simulink model "p2a"  (R2017b)
settings: Solver=FixedStepAuto  StartTime=0.0  StopTime=10.0  FixedStep=0.01  RelTol=1e-3
values from neighbouring files (symbols this model uses):
  a = [ -0.0000 1.0000 -0.0000 -0.0000 ... (first row only)    [observer.m]    (also in p2a.m)
  b = [ -0.0000 0.0000 ... (first row only)    [observer.m]    (also in p2a.m)
  c = [ 1.0000 -0.0050 0.0000 0.0000 ... (first row only)    [observer.m]    (also in p2a.m)
undefined symbols (not defined in the file or in its folder): K, l1
settings Model: Creator=Soutrik  LastModifiedBy=Soutrik

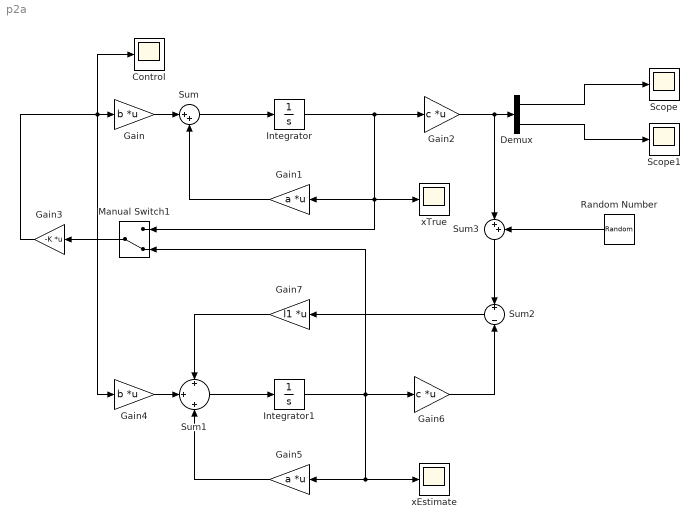
== system p2a ==
  Control : Scope
  Demux : Demux  Outputs=2
  Gain : Gain  Gain=b  Multiplication=Matrix(K*u)
  Gain1 : Gain  Gain=a  Multiplication=Matrix(K*u)
  Gain2 : Gain  Gain=c  Multiplication=Matrix(K*u)
  Gain3 : Gain  Gain=-K  Multiplication=Matrix(K*u)
  Gain4 : Gain  Gain=b  Multiplication=Matrix(K*u)
  Gain5 : Gain  Gain=a  Multiplication=Matrix(K*u)
  Gain6 : Gain  Gain=c  Multiplication=Matrix(K*u)
  Gain7 : Gain  Gain=l1  Multiplication=Matrix(K*u)
  Integrator : Integrator  InitialCondition=[0.05, 0, 0, 0]
  Integrator1 : Integrator  InitialCondition=[0.05, 0, 0, 0]
  Manual Switch1 : ManualSwitch  CurrentSetting=0
  Random Number : RandomNumber  Variance=[0.00001, 0.00001, 0.0001, 0.0001]  Seed=[1 2 3 4]  SampleTime=0.01
  Scope : Scope
  Scope1 : Scope
  Sum : Sum  Inputs=|++
  Sum1 : Sum  Inputs=+|+|+
  Sum2 : Sum  Inputs=+||-
  Sum3 : Sum  Inputs=|++
  xEstimate : Scope
  xTrue : Scope
  wires:
  Random Number/1 -> Sum3/2
  Gain7/1 -> Sum1/1
  Sum3/1 -> Sum2/1
  Manual Switch1/1 -> Gain3/1
  Gain2/1 -> Sum3/1, Demux/1
  Gain5/1 -> Sum1/3
  Gain6/1 -> Sum2/2
  Sum1/1 -> Integrator1/1
  Gain4/1 -> Sum1/2
  Gain1/1 -> Sum/2
  Integrator1/1 -> Manual Switch1/2, Gain6/1, xEstimate/1, Gain5/1
  Demux/2 -> Scope1/1
  Sum/1 -> Integrator/1
  Gain3/1 -> Gain4/1, Control/1, Gain/1
  Gain/1 -> Sum/1
  Demux/1 -> Scope/1
  Sum2/1 -> Gain7/1
  Integrator/1 -> Manual Switch1/1, xTrue/1, Gain1/1, Gain2/1
